simulink model "laba1"  (R2023a)
settings: Solver=VariableStepAuto  StartTime=0.0  StopTime=3  RelTol=1e-3
values from neighbouring files (symbols this model uses):
  Betta = 0.001    [script1.m]
  CM = 1.3    [script1.m]
  COm = 3.15    [script1.m]
  Jdv = 7e-6    (= 7e-06)    [script1.m]
  Lob = 0.013    [script1.m]
  Ly = 0.0015    [script1.m]
  R = 8    [script1.m]
settings Model: Creator=kwabo  LastModifiedBy=kwabo

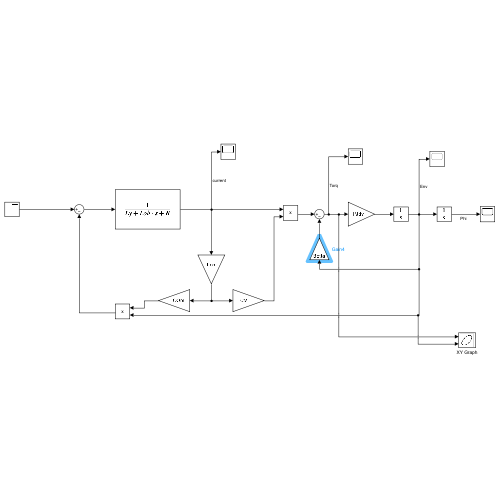
[thumbnail: Simulink's stored preview of the top-level diagram]
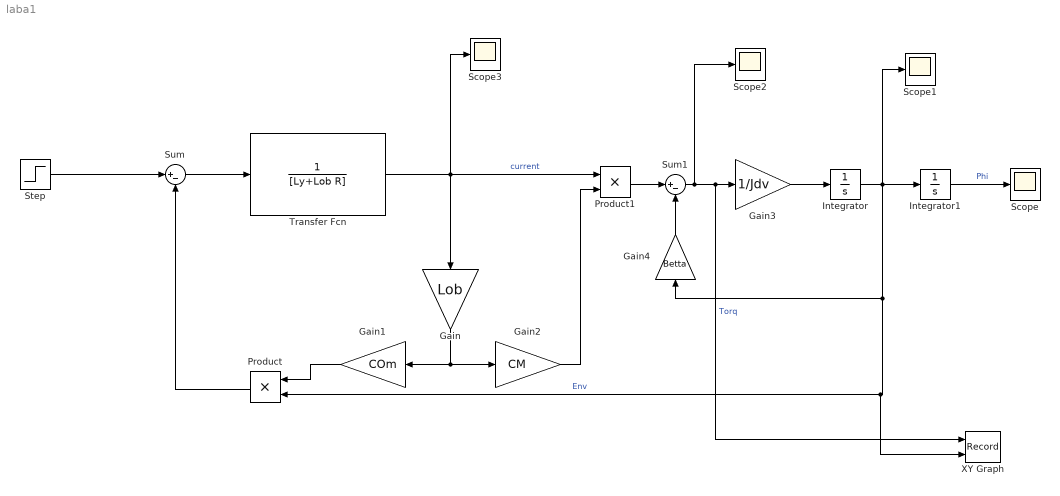
== system laba1 ==
  Gain : Gain  Gain=Lob
  Gain1 : Gain  Gain=COm
  Gain2 : Gain  Gain=CM
  Gain3 : Gain  Gain=1/Jdv
  Gain4 : Gain  Gain=Betta
  Integrator : Integrator
  Integrator1 : Integrator
  Product : Product
  Product1 : Product
  Scope{,1..3} (4 alike) : Scope
  Step : Step  Time=0  After=10  SampleTime=0
  Sum : Sum  Inputs=|+-
  Sum1 : Sum  Inputs=|+-
  Transfer Fcn : TransferFcn  Denominator=[Ly+Lob R]
  XY Graph : Record  FileSettingsInternal="{\"entries\":[{\"content\":{\"excelSettings\":{\"content\":{},\"type\":\"Streamout.ExcelSettings\"}},\"type\":\"Streamout.FileSettingStorage\",\"uuid\":\"0fca94d6-95ea-4c8f-bf67-0a1f5e900f40\"}],\"packageUris\":[\"http://schema.mathworks.com/mf0/streamout_blocks/R2020a\"],\"version\":\"1.0\"}"  Layout=[1 1]  SignalsInternal="{\"entries\":[{\"content\":{\"signals\":[{\"content\":{\"blockPath\":[\"untitled/XY Graph\"],\"dimensions\":[1],\"domain\":\"untitled/XY Graph\",\"lineColor\":\"#a2142f\",\"port\":1,\"sid\":[\"\"],\"signalID\":213,\"signalName\":\"Torq\"},\"type\":\"RecordBlkView.Signal\",\"uuid\":\"1a6f5d1e-8195-4029-87ff-375a8f96fe9b\"},{\"content\":{\"blockPath\":[\"untitled/XY Graph\"],\"dimensions\":[1],\"domain\":\"untitled/XY Graph\",\"lineColor\":\"#139fff\",\"port\":2,\"sid\":[\"\"],\"signalID\":217,\"signalName\":\"Env\"},\"type\":\"RecordBlkView.Signal\",\"uuid\":\"d07f0591-5891-4efc-808f-81e57299092d\"}]},\"type\":\"RecordBlkView.InputSignals\",\"uuid\":\"98226874-f521-40eb-9a15-09d4be935fae\"}],\"packageUris\":[\"http://schema.mathworks.com/mf0/streamout_blocks/R2020a\"],\"version\":\"1.0\"}"  VisualizationBindings="{\"xyplotplugin\":{\"info\":[{\"series\":[{\"bindingParametersList\":[{\"parameter\":\"X-Axis\",\"signalID\":158,\"signalName\":\"Env\"},{\"parameter\":\"Y-Axis\",\"signalID\":154,\"signalName\":\"Torq\"}],\"seriesID\":34083}],\"subplotID\":1}]}}"  CompatibilityTag=XY
  wires:
  Transfer Fcn/1 -> Scope3/1, Product1/1, Gain/1  "current"
  Gain/1 -> Gain2/1, Gain1/1
  Gain1/1 -> Product/1
  Sum/1 -> Transfer Fcn/1
  Product/1 -> Sum/2
  Gain2/1 -> Product1/2
  Product1/1 -> Sum1/1
  Gain4/1 -> Sum1/2
  Sum1/1 -> Scope2/1, XY Graph/1, Gain3/1  "Torq"
  Gain3/1 -> Integrator/1
  Integrator/1 -> Scope1/1, Gain4/1, XY Graph/2, Product/2, Integrator1/1  "Env"
  Integrator1/1 -> Scope/1  "Phi"
  Step/1 -> Sum/1
